simulink model "StateFeedbackDraft"  (R2023a)
settings: Solver=VariableStepAuto  StartTime=0.0  StopTime=10.0  RelTol=1e-3
settings Model: Creator=19591  LastModifiedBy=19591

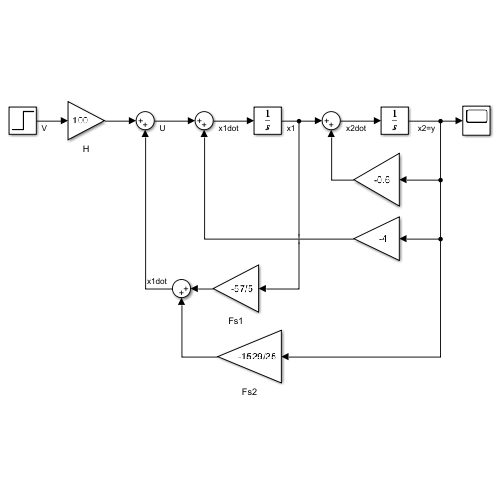
[thumbnail: Simulink's stored preview of the top-level diagram]
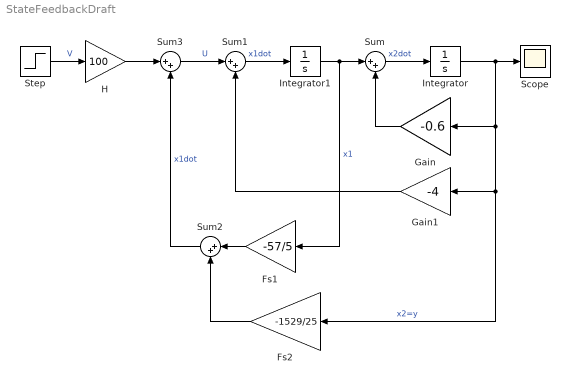
== system StateFeedbackDraft ==
  Fs1 : Gain  Gain=-57/5
  Fs2 : Gain  Gain=-1529/25
  Gain : Gain  Gain=-0.6
  Gain1 : Gain  Gain=-4
  H : Gain  Gain=100
  Integrator : Integrator
  Integrator1 : Integrator
  Scope : Scope
  Step : Step  SampleTime=0
  Sum{,1..3} (4 alike) : Sum  Inputs=|++
  wires:
  Integrator/1 -> Fs2/1, Gain1/1, Gain/1, Scope/1  "x2=y"
  Gain/1 -> Sum/2
  Sum/1 -> Integrator/1  "x2dot"
  Integrator1/1 -> Fs1/1, Sum/1  "x1"
  Sum1/1 -> Integrator1/1  "x1dot"
  Gain1/1 -> Sum1/2
  Fs1/1 -> Sum2/1
  Fs2/1 -> Sum2/2
  Sum3/1 -> Sum1/1  "U"
  Step/1 -> H/1  "V"
  Sum2/1 -> Sum3/2  "x1dot"
  H/1 -> Sum3/1
